simulink model "InertialMeasurementUnit_model"  (R2015a)
settings: Solver=ode45  StartTime=0.0  StopTime=10.0  RelTol=1e-3
settings Model: Creator=hamada  LastModifiedBy=hamada

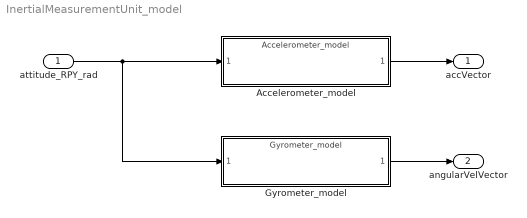
== system InertialMeasurementUnit_model ==
  attitude_RPY_rad : Inport  PortDimensions=3
  Accelerometer_model : ModelReference  ModelNameDialog=Accelerometer_model.slx  SimulationMode=Normal  ModelReferenceVersion=1.10  CopyOfModelName=Accelerometer_model.slx  DefaultDataLogging=on
  Gyrometer_model : ModelReference  ModelNameDialog=Gyrometer_model.slx  SimulationMode=Normal  ModelReferenceVersion=1.12  CopyOfModelName=Gyrometer_model.slx  DefaultDataLogging=on
  accVector : Outport
  angularVelVector : Outport  Port=2
  wires:
  Accelerometer_model/1 -> accVector/1
  Gyrometer_model/1 -> angularVelVector/1
  attitude_RPY_rad/1 -> Accelerometer_model/1, Gyrometer_model/1
